simulink model "SVF"  (R2021a)
settings: Solver=VariableStepAuto  StartTime=0.0  StopTime=10.0  RelTol=1e-3
libraries: audiosources x6
settings Model: Creator=Asurans  LastModifiedBy=Asurans

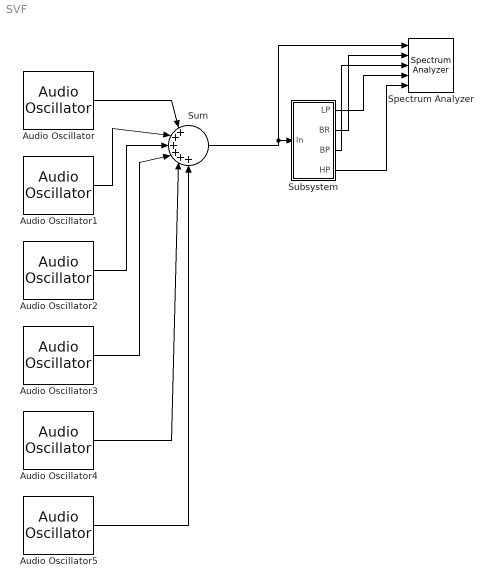
== system SVF ==
  Audio Oscillator : audiosources/Audio Oscillator  FrequencyPort=off  Frequency=50  AmplitudePort=off  Amplitude=32000  DCOffsetPort=off  PhaseOffset=0  DCOffset=0  WidthPort=off  Width=1  DutyCyclePort=off  DutyCycle=0.5  SampsPerFrame=2500  Fs=48000  OutputDataType=single  SimulateUsing=Code generation
      settings: SourceProductBaseCode=AU  SignalType=sine
  Audio Oscillator1 : audiosources/Audio Oscillator  FrequencyPort=off  Frequency=80  AmplitudePort=off  Amplitude=32000  DCOffsetPort=off  PhaseOffset=0  DCOffset=0  WidthPort=off  Width=1  DutyCyclePort=off  DutyCycle=0.5  SampsPerFrame=2500  Fs=48000  OutputDataType=single  SimulateUsing=Code generation
      settings: SourceProductBaseCode=AU  SignalType=sine
  Audio Oscillator2 : audiosources/Audio Oscillator  FrequencyPort=off  Frequency=100  AmplitudePort=off  Amplitude=32000  DCOffsetPort=off  PhaseOffset=0  DCOffset=0  WidthPort=off  Width=1  DutyCyclePort=off  DutyCycle=0.5  SampsPerFrame=2500  Fs=48000  OutputDataType=single  SimulateUsing=Code generation
      settings: SourceProductBaseCode=AU  SignalType=sine
  Audio Oscillator3 : audiosources/Audio Oscillator  FrequencyPort=off  Frequency=200  AmplitudePort=off  Amplitude=32000  DCOffsetPort=off  PhaseOffset=0  DCOffset=0  WidthPort=off  Width=1  DutyCyclePort=off  DutyCycle=0.5  SampsPerFrame=2500  Fs=48000  OutputDataType=single  SimulateUsing=Code generation
      settings: SourceProductBaseCode=AU  SignalType=sine
  Audio Oscillator4 : audiosources/Audio Oscillator  FrequencyPort=off  Frequency=500  AmplitudePort=off  Amplitude=32000  DCOffsetPort=off  PhaseOffset=0  DCOffset=0  WidthPort=off  Width=1  DutyCyclePort=off  DutyCycle=0.5  SampsPerFrame=2500  Fs=48000  OutputDataType=single  SimulateUsing=Code generation
      settings: SourceProductBaseCode=AU  SignalType=sine
  Audio Oscillator5 : audiosources/Audio Oscillator  FrequencyPort=off  Frequency=1000  AmplitudePort=off  Amplitude=32000  DCOffsetPort=off  PhaseOffset=0  DCOffset=0  WidthPort=off  Width=1  DutyCyclePort=off  DutyCycle=0.5  SampsPerFrame=2500  Fs=48000  OutputDataType=single  SimulateUsing=Code generation
      settings: SourceProductBaseCode=AU  SignalType=sine
  Spectrum Analyzer : SpectrumAnalyzer  NumInputPorts=5
  Subsystem : Subsystem
  Sum : Sum  Inputs=|++++++
  wires:
  Subsystem/1(LP) -> Spectrum Analyzer/4
  Subsystem/4(HP) -> Spectrum Analyzer/5
  Subsystem/2(BR) -> Spectrum Analyzer/2
  Subsystem/3(BP) -> Spectrum Analyzer/3
  Sum/1 -> Spectrum Analyzer/1, Subsystem/1(In)
  Audio Oscillator/1 -> Sum/1
  Audio Oscillator1/1 -> Sum/2
  Audio Oscillator2/1 -> Sum/3
  Audio Oscillator3/1 -> Sum/4
  Audio Oscillator4/1 -> Sum/5
  Audio Oscillator5/1 -> Sum/6

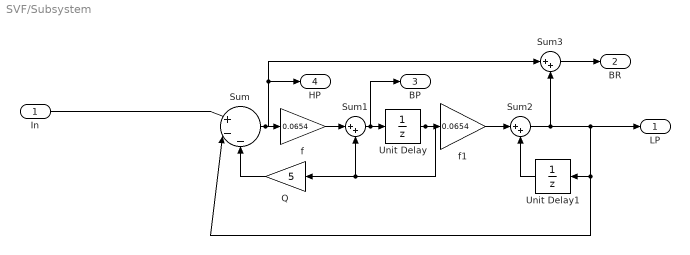
== system SVF/Subsystem ==
  In : Inport
  Q : Gain  Gain=5
  Sum : Sum  Inputs=|+--
  Sum1 : Sum  Inputs=|++
  Sum2 : Sum  Inputs=|++
  Sum3 : Sum  Inputs=|++
  Unit Delay : UnitDelay  SampleTime=-1  HasFrameUpgradeWarning=on
  Unit Delay1 : UnitDelay  SampleTime=-1  HasFrameUpgradeWarning=on
  f : Gain  Gain=0.0654
  f1 : Gain  Gain=0.0654
  LP : Outport
  BR : Outport  Port=2
  BP : Outport  Port=3
  HP : Outport  Port=4
  wires:
  Unit Delay/1 -> Q/1, Sum1/2, f1/1
  Sum/1 -> HP/1, Sum3/1, f/1
  Sum3/1 -> BR/1
  Sum2/1 -> Sum3/2, LP/1, Sum/2, Unit Delay1/1
  f1/1 -> Sum2/1
  Q/1 -> Sum/3
  Unit Delay1/1 -> Sum2/2
  f/1 -> Sum1/1
  Sum1/1 -> BP/1, Unit Delay/1
  In/1 -> Sum/1
